simulink model "tallerpto3"  (R2021a)
settings: Solver=VariableStepAuto  StartTime=0.0  StopTime=1.7  RelTol=1e-3
settings Model: Creator=retou  LastModifiedBy=retou
settings SolverCC: AlgebraicLoopSolver=TrustRegion
settings DebuggingCC: SFMachineParentedDataDiag=warning

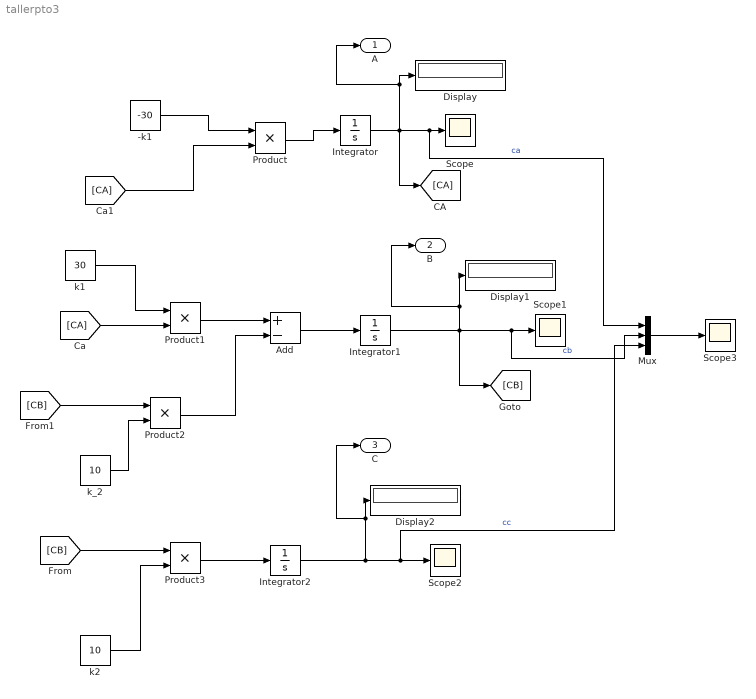
== system tallerpto3 ==
  -k1 : Constant  Value=-30
  Add : Sum  Inputs=+-
  Display : Display
  Display1 : Display
  Display2 : Display
  Integrator : Integrator  InitialCondition=100
  Integrator1 : Integrator
  Integrator2 : Integrator
  Mux : Mux  Inputs=3
  Product{,1..3} (4 alike) : Product
  Scope{,1..3} (4 alike) : Scope
  k1 : Constant  Value=30
  k2 : Constant  Value=10
  k_2 : Constant  Value=10
  A : Outport
  B : Outport  Port=2
  C : Outport  Port=3
  wires:
  [CA] -> Product/2
  -k1/1 -> Product/1
  Product/1 -> Integrator/1
  Integrator/1 -> A/1, Display/1, [CA], Mux/1, Scope/1  "ca"
  [CA] -> Product1/2
  k1/1 -> Product1/1
  Product1/1 -> Add/1
  [CB] -> Product2/1
  k_2/1 -> Product2/2
  Product2/1 -> Add/2
  Add/1 -> Integrator1/1
  Integrator1/1 -> B/1, Display1/1, [CB], Mux/2, Scope1/1  "cb"
  [CB] -> Product3/1
  k2/1 -> Product3/2
  Product3/1 -> Integrator2/1
  Mux/1 -> Scope3/1
  Integrator2/1 -> Mux/3, Scope2/1, C/1, Display2/1  "cc"
